simulink model "hclab7"  (Simulink 7.7)
settings: Solver=ode45  StartTime=0.0  StopTime=20  RelTol=1e-3
settings Model: Creator=student  LastModifiedBy=mestan

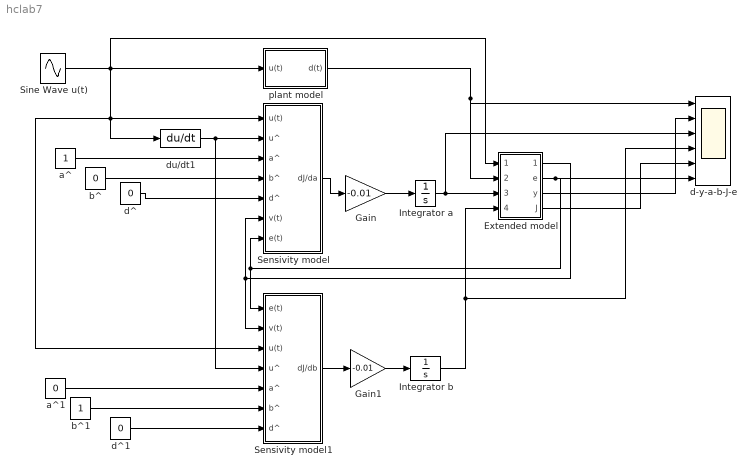
== system hclab7 ==
  Extended model : Subsystem
  Gain : Gain  Gain=-0.01
  Gain1 : Gain  Gain=-0.01
  Integrator a : Integrator
  Integrator b : Integrator
  Sensivity model : Subsystem
  Sensivity model1 : Subsystem
  Sine Wave u(t) : Sin  Amplitude=3  Frequency=50  SampleTime=0
  a^ : Constant
  a^1 : Constant  Value=0
  b^ : Constant  Value=0
  b^1 : Constant
  d-y-a-b-J-e : Scope  NumInputPorts=6
      settings: TimeRange=10  YMin=-0.5~-0.15~-5.55112e-017~-5.55112e-017~-1.38778e-017~-0.6  YMax=0.6~0.15~0.7~0.7~0.175~0.4
  d^ : Constant  Value=0
  d^1 : Constant  Value=0
  du/dt1 : Derivative
  plant model : Subsystem
  wires:
  Gain1/1 -> Integrator b/1
  Gain/1 -> Integrator a/1
  Sensivity model/1(dJ/da) -> Gain/1
  Sine Wave u(t)/1 -> plant model/1(u(t)), du/dt1/1, Sensivity model/1(u(t)), Sensivity model1/3(u(t)), Extended model/1(u(t))
  du/dt1/1 -> Sensivity model/2(u^), Sensivity model1/4(u^)
  a^/1 -> Sensivity model/3(a^)
  b^/1 -> Sensivity model/4(b^)
  d^/1 -> Sensivity model/5(d^)
  a^1/1 -> Sensivity model1/5(a^)
  b^1/1 -> Sensivity model1/6(b^)
  d^1/1 -> Sensivity model1/7(d^)
  Sensivity model1/1(dJ/db) -> Gain1/1
  plant model/1(d(t)) -> Extended model/2(d(t)), d-y-a-b-J-e/1
  Integrator a/1 -> d-y-a-b-J-e/3, Extended model/3(a(t))
  Integrator b/1 -> Extended model/4(b(t)), d-y-a-b-J-e/4
  Extended model/2(e) -> Sensivity model/7(e(t)), Sensivity model1/1(e(t)), d-y-a-b-J-e/6
  Extended model/1(v(t)) -> Sensivity model/6(v(t)), Sensivity model1/2(v(t))
  Extended model/4(J) -> d-y-a-b-J-e/5
  Extended model/3(y) -> d-y-a-b-J-e/2

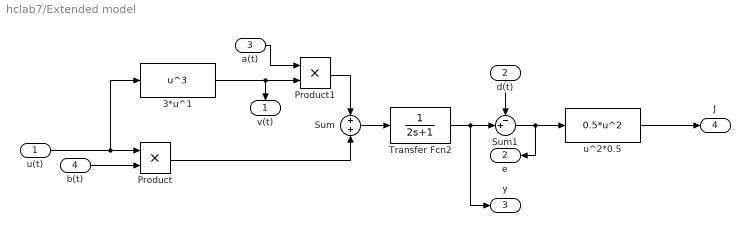
== system hclab7/Extended model ==
  u(t) : Inport
  d(t) : Inport  Port=2
  a(t) : Inport  Port=3
  b(t) : Inport  Port=4
  3*u^1 : MATLABFcn  MATLABFcn=u^3
  Product : Product  RndMeth=Zero
  Product1 : Product  RndMeth=Zero
  Sum : Sum  Inputs=+|+
  Sum1 : Sum  Inputs=-+|
  Transfer Fcn2 : TransferFcn  Denominator=[2 1]
  u^2*0.5 : MATLABFcn  MATLABFcn=0.5*u^2
  v(t) : Outport
  e : Outport  Port=2
  y : Outport  Port=3
  J : Outport  Port=4
  wires:
  3*u^1/1 -> Product1/2, v(t)/1
  Sum/1 -> Transfer Fcn2/1
  Product1/1 -> Sum/1
  Product/1 -> Sum/2
  Transfer Fcn2/1 -> Sum1/2, y/1
  Sum1/1 -> e/1, u^2*0.5/1
  a(t)/1 -> Product1/1
  d(t)/1 -> Sum1/1
  u(t)/1 -> Product/1, 3*u^1/1
  b(t)/1 -> Product/2
  u^2*0.5/1 -> J/1

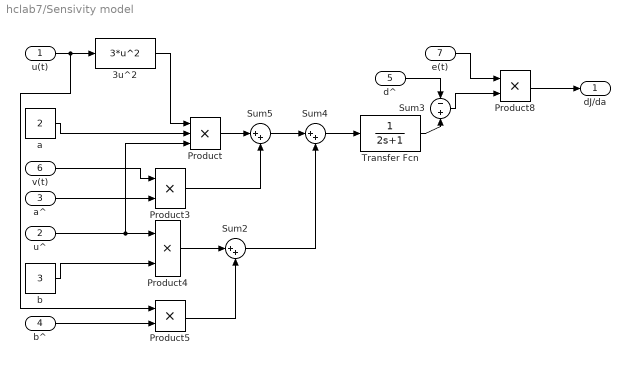
== system hclab7/Sensivity model ==
  u(t) : Inport
  u^ : Inport  Port=2
  a^ : Inport  Port=3
  b^ : Inport  Port=4
  d^ : Inport  Port=5
  v(t) : Inport  Port=6
  e(t) : Inport  Port=7
  3u^2 : MATLABFcn  MATLABFcn=3*u^2
  Product : Product  Inputs=3  RndMeth=Zero
  Product{3..5,8} (4 alike) : Product  RndMeth=Zero
  Sum2 : Sum  Inputs=|++
  Sum3 : Sum  Inputs=-|+
  Sum4 : Sum  Inputs=|++
  Sum5 : Sum  Inputs=|++
  Transfer Fcn : TransferFcn  Denominator=[2 1]
  a : Constant  Value=2
  b : Constant  Value=3
  dJ/da : Outport
  wires:
  u(t)/1 -> 3u^2/1, Product5/1
  a^/1 -> Product3/2
  b^/1 -> Product5/2
  Product5/1 -> Sum2/2
  Transfer Fcn/1 -> Sum3/2
  d^/1 -> Sum3/1
  Sum3/1 -> Product8/2
  u^/1 -> Product4/1, Product/3
  b/1 -> Product4/2
  Product4/1 -> Sum2/1
  a/1 -> Product/2
  3u^2/1 -> Product/1
  v(t)/1 -> Product3/1
  Product/1 -> Sum5/1
  Product3/1 -> Sum5/2
  Sum5/1 -> Sum4/1
  Sum2/1 -> Sum4/2
  Sum4/1 -> Transfer Fcn/1
  e(t)/1 -> Product8/1
  Product8/1 -> dJ/da/1

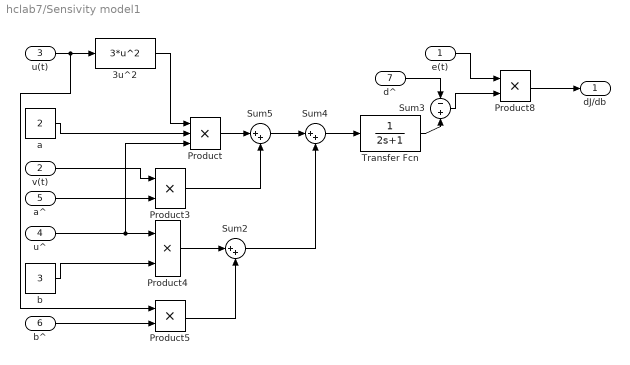
== system hclab7/Sensivity model1 ==
  e(t) : Inport
  v(t) : Inport  Port=2
  u(t) : Inport  Port=3
  u^ : Inport  Port=4
  a^ : Inport  Port=5
  b^ : Inport  Port=6
  d^ : Inport  Port=7
  3u^2 : MATLABFcn  MATLABFcn=3*u^2
  Product : Product  Inputs=3  RndMeth=Zero
  Product{3..5,8} (4 alike) : Product  RndMeth=Zero
  Sum2 : Sum  Inputs=|++
  Sum3 : Sum  Inputs=-|+
  Sum4 : Sum  Inputs=|++
  Sum5 : Sum  Inputs=|++
  Transfer Fcn : TransferFcn  Denominator=[2 1]
  a : Constant  Value=2
  b : Constant  Value=3
  dJ/db : Outport
  wires:
  u(t)/1 -> 3u^2/1, Product5/1
  a^/1 -> Product3/2
  b^/1 -> Product5/2
  Product5/1 -> Sum2/2
  Transfer Fcn/1 -> Sum3/2
  d^/1 -> Sum3/1
  Sum3/1 -> Product8/2
  u^/1 -> Product4/1, Product/3
  b/1 -> Product4/2
  Product4/1 -> Sum2/1
  a/1 -> Product/2
  3u^2/1 -> Product/1
  v(t)/1 -> Product3/1
  Product/1 -> Sum5/1
  Product3/1 -> Sum5/2
  Sum5/1 -> Sum4/1
  Sum2/1 -> Sum4/2
  Sum4/1 -> Transfer Fcn/1
  e(t)/1 -> Product8/1
  Product8/1 -> dJ/db/1

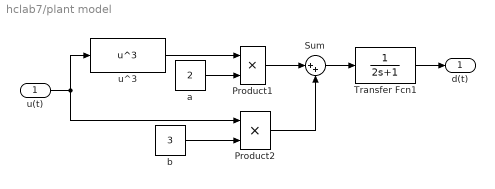
== system hclab7/plant model ==
  u(t) : Inport
  Product1 : Product  RndMeth=Zero
  Product2 : Product  RndMeth=Zero
  Sum : Sum  Inputs=|++
  Transfer Fcn1 : TransferFcn  Denominator=[2 1]
  a : Constant  Value=2
  b : Constant  Value=3
  u^3 : MATLABFcn  MATLABFcn=u^3
  d(t) : Outport
  wires:
  u(t)/1 -> u^3/1, Product2/1
  b/1 -> Product2/2
  u^3/1 -> Product1/1
  a/1 -> Product1/2
  Product1/1 -> Sum/1
  Product2/1 -> Sum/2
  Sum/1 -> Transfer Fcn1/1
  Transfer Fcn1/1 -> d(t)/1
